simulink model "BLDC_Motor"  (R2018b)
settings: Solver=FixedStepDiscrete  StartTime=0.0  StopTime=2  MaxStep=1e-4  RelTol=1e-4
values from neighbouring files (symbols this model uses):
  A = 0    [control.m]
libraries: powerlib x10
settings Model: Creator=Nick  LastModifiedBy=Nick
settings SFSimCC: SimUseLocalCustomCode=off
settings RTWCC: RTWUseLocalCustomCode=off
settings CodeAppCC: StateflowObjectComments=on

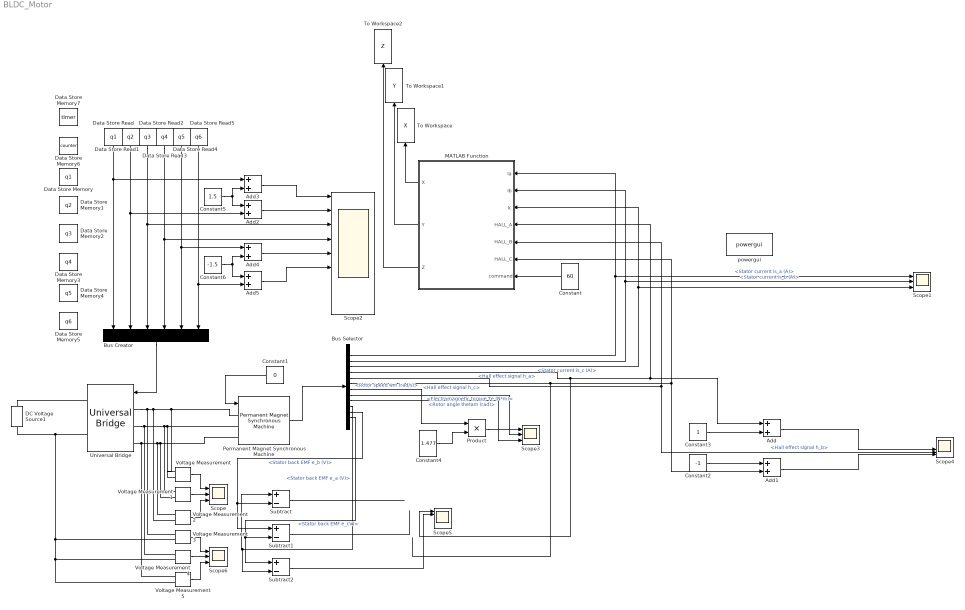
== system BLDC_Motor ==
  Add{,1..5} (6 alike) : Sum
  Bus Creator : BusCreator  Inputs=6
  Bus Selector : BusSelector  OutputSignals=Stator current is_a (A),Stator current is_b (A),Stator current is_c (A),Hall effect signal h_a,Hall effect signal h_b,Hall effect signal h_c,Rotor speed wm (rad/s),Electromagnetic torque Te (N*m),Rotor angle thetam (rad),Stator back EMF e_a (V),Stator back EMF e_b (V),Stator back EMF e_cV)
  Constant : Constant  Value=60
  Constant1 : Constant  Value=0
  Constant2 : Constant  Value=-1
  Constant3 : Constant
  Constant4 : Constant  Value=1.477
  Constant5 : Constant  Value=1.5
  Constant6 : Constant  Value=-1.5
  DC Voltage Source1 : powerlib/Electrical Sources/DC Voltage Source  Amplitude=48  Measurements=None
      settings: SourceProductName=Simscape Electrical
  Data Store Memory : DataStoreMemory  DataStoreName=q1  ReadBeforeWriteMsg=warning  WriteAfterWriteMsg=warning  WriteAfterReadMsg=warning  ShowAdditionalParam=off  OutDataTypeStr=double
  Data Store Memory1 : DataStoreMemory  DataStoreName=q2  ReadBeforeWriteMsg=warning  WriteAfterWriteMsg=warning  WriteAfterReadMsg=warning  ShowAdditionalParam=off  OutDataTypeStr=double
  Data Store Memory2 : DataStoreMemory  DataStoreName=q3  ReadBeforeWriteMsg=warning  WriteAfterWriteMsg=warning  WriteAfterReadMsg=warning  ShowAdditionalParam=off  OutDataTypeStr=double
  Data Store Memory3 : DataStoreMemory  DataStoreName=q4  ReadBeforeWriteMsg=warning  WriteAfterWriteMsg=warning  WriteAfterReadMsg=warning  ShowAdditionalParam=off  OutDataTypeStr=double
  Data Store Memory4 : DataStoreMemory  DataStoreName=q5  ReadBeforeWriteMsg=warning  WriteAfterWriteMsg=warning  WriteAfterReadMsg=warning  ShowAdditionalParam=off  OutDataTypeStr=double
  Data Store Memory5 : DataStoreMemory  DataStoreName=q6  ReadBeforeWriteMsg=warning  WriteAfterWriteMsg=warning  WriteAfterReadMsg=warning  ShowAdditionalParam=off  OutDataTypeStr=double
  Data Store Memory6 : DataStoreMemory  DataStoreName=counter  ReadBeforeWriteMsg=warning  WriteAfterWriteMsg=warning  WriteAfterReadMsg=warning  ShowAdditionalParam=off  OutDataTypeStr=double
  Data Store Memory7 : DataStoreMemory  DataStoreName=timer  ReadBeforeWriteMsg=warning  WriteAfterWriteMsg=warning  WriteAfterReadMsg=warning  ShowAdditionalParam=off  OutDataTypeStr=double
  Data Store Read : DataStoreRead  DataStoreName=q1
  Data Store Read1 : DataStoreRead  DataStoreName=q2
  Data Store Read2 : DataStoreRead  DataStoreName=q3
  Data Store Read3 : DataStoreRead  DataStoreName=q4
  Data Store Read4 : DataStoreRead  DataStoreName=q5
  Data Store Read5 : DataStoreRead  DataStoreName=q6
  MATLAB Function : MATLAB Function  TreatAsAtomicUnit=on
  Permanent Magnet Synchronous Machine : powerlib/Machines/Permanent Magnet Synchronous Machine  NbPhases=3  FluxDistribution=Trapezoidal  RotorType=Round  MechanicalLoad=Torque Tm  PresetModel=No  ShowDetailedParameters=on  MeasurementBus=off  Resistance=0.0485  Inductance=8.5e-3  dqInductances=[8.5e-3,8.5e-3]  La=0.000395  MachineConstant=Flux linkage established by magnets (V.s)  Flux=0.1194  VoltageCst=100.0283  TorqueCst=0.9552  Flat=120  Mechanical=[0.0027 0.0004924 4 0]  PolePairs=4  InitialConditions=[0,0, 0,0]  InitialConditions5ph=[0 0 0 0 0 0]  TsPowergui=0  TsBlock=-1  RefAngle=90 degrees behind phase A axis (modified Park)
  Product : Product
  Scope{,1,3,6} (4 alike) : Scope  NumInputPorts=3
  Scope2 : Scope  NumInputPorts=9
  Scope4 : Scope  NumInputPorts=6
  Scope5 : Scope  NumInputPorts=6
  Subtract : Sum  Inputs=+-
  Subtract1 : Sum  Inputs=+-
  Subtract2 : Sum  Inputs=+-
  To Workspace : ToWorkspace  VariableName=X  SaveFormat=Timeseries  SampleTime=-1
  To Workspace1 : ToWorkspace  VariableName=Y  SaveFormat=Timeseries  SampleTime=-1
  To Workspace2 : ToWorkspace  VariableName=Z  SaveFormat=Timeseries  SampleTime=-1
  Universal Bridge : powerlib/Power Electronics/Universal Bridge  Arms=3  SnubberResistance=1e5  SnubberCapacitance=inf  Device=MOSFET / Diodes  Ron=1e-3  Lon=0  ForwardVoltages="[  0  0  ]"  ForwardVoltage=0  GTOparameters=[ 10e-6 , 20e-6 ]  IGBTparameters=[ 1e-6 , 2e-6 ]  Measurements=None  Measurements_2=None  converterType=Rectifier
      settings: SourceProductName=Simscape Electrical
  Voltage Measurement{,1..5} (6 alike) : powerlib/Measurements/Voltage Measurement  PhasorSimulation=off  OutputType=Complex  PSBequivalent=0
      settings: SourceProductName=Simscape Electrical
  powergui : powerlib/powergui  Priority=1  SimulationMode=Discrete  SampleTime=50e-6  frequency=60  Iterations=50  frequencyindice=0  Pbase=100e6  ErrMax=1e-4  UnitsV=kV  UnitsW=MW  buscounter=0  FunctionMessages=off  echomessages=off  EnableUseOfTLC=off  CurrentSourceSwitches=off  DisableSnubberDevices=off  DisableRonSwitches=off  DisableVfSwitches=off  DisplayEquations=off  SolverType=Tustin/Backward Euler (TBE)  Interpol=off  ExternalGateDelay=off  methode=off  Ts=100  x0status=blocks  SPID=off  SwTol=0  HookPort=off  RestoreLinks=warning  ResistiveCurrentMeasurement=off  Frange=[0:2:500]  Ylog=off  Xlog=on  ShowGrid=off  save=off  variable=ZData  structure=0  ZoomFFT=off  StartTime=0.0  cycles=1  DisplayStyle=1  fundamental=60  FreqAxis=off  MaxFrequency=1000  frequencyindicesteady=1  RmsSteady=1  display=off
      settings: SourceProductName=Simscape Electrical
  wires:
  Permanent Magnet Synchronous Machine/1 -> Bus Selector/1
  Bus Selector/1 -> Scope1/1, MATLAB Function/1(Ia)  "<Stator current is_a (A)>"
  Constant/1 -> MATLAB Function/7(command)
  Bus Selector/2 -> Scope1/2, MATLAB Function/2(Ib)  "<Stator current is_b (A)>"
  Bus Selector/3 -> Scope1/3, MATLAB Function/3(Ic)  "<Stator current is_c (A)>"
  Bus Selector/5 -> Scope4/5, MATLAB Function/5(HALL_B)  "<Hall effect signal h_b>"
  Bus Selector/6 -> Add1/2, MATLAB Function/6(HALL_C)  "<Hall effect signal h_c>"
  Bus Selector/4 -> Scope5/1, Add/1, MATLAB Function/4(HALL_A)  "<Hall effect signal h_a>"
  Voltage Measurement/1 -> Scope/1
  Bus Creator/1 -> Universal Bridge/1
  Constant3/1 -> Add/2
  Constant2/1 -> Add1/1
  Add1/1 -> Scope4/6
  Add/1 -> Scope4/4
  Data Store Read/1 -> Bus Creator/1, Add3/1
  Data Store Read2/1 -> Scope2/3, Bus Creator/3
  Data Store Read3/1 -> Scope2/4, Bus Creator/4
  Data Store Read4/1 -> Add4/1, Bus Creator/5
  Constant1/1 -> Permanent Magnet Synchronous Machine/1
  Bus Selector/7 -> Product/1  "<Rotor speed wm (rad/s)>"
  Constant4/1 -> Product/2
  Product/1 -> Scope3/1
  Voltage Measurement4/1 -> Scope6/2
  Voltage Measurement3/1 -> Scope6/1
  Voltage Measurement5/1 -> Scope6/3
  Data Store Read1/1 -> Add2/2, Bus Creator/2
  Bus Selector/8 -> Scope3/2  "<Electromagnetic torque Te (N*m)>"
  Bus Selector/9 -> Scope3/3  "<Rotor angle thetam (rad)>"
  Voltage Measurement1/1 -> Scope/2
  Voltage Measurement2/1 -> Scope/3
  Add2/1 -> Scope2/2
  Constant5/1 -> Add2/1, Add3/2
  Add3/1 -> Scope2/1
  Add4/1 -> Scope2/5
  Add5/1 -> Scope2/6
  Constant6/1 -> Add5/1, Add4/2
  Data Store Read5/1 -> Add5/2, Bus Creator/6
  MATLAB Function/1(X) -> To Workspace/1
  MATLAB Function/2(Y) -> To Workspace1/1
  MATLAB Function/3(Z) -> To Workspace2/1
  Bus Selector/11 -> Subtract/2, Subtract1/1  "<Stator back EMF e_b (V)>"
  Subtract/1 -> ?
  Bus Selector/12 -> Subtract2/1, Subtract1/2  "<Stator back EMF e_cV)>"
  Bus Selector/10 -> Subtract2/2, Subtract/1  "<Stator back EMF e_a (V)>"
  Subtract1/1 -> ?
  Subtract2/1 -> Scope5/2
  connections:
  Universal Bridge/LConn1 -- Voltage Measurement3/LConn1 -- Voltage Measurement2/LConn2 -- Permanent Magnet Synchronous Machine/LConn1 -- Voltage Measurement/LConn1
  Universal Bridge/LConn2 -- Voltage Measurement4/LConn1 -- Voltage Measurement1/LConn1 -- Permanent Magnet Synchronous Machine/LConn2 -- Voltage Measurement/LConn2
  Universal Bridge/LConn3 -- Voltage Measurement5/LConn1 -- Voltage Measurement2/LConn1 -- Permanent Magnet Synchronous Machine/LConn3 -- Voltage Measurement1/LConn2
  Universal Bridge/RConn1 -- DC Voltage Source1/RConn1
  Universal Bridge/RConn2 -- Voltage Measurement5/LConn2 -- Voltage Measurement4/LConn2 -- Voltage Measurement3/LConn2 -- DC Voltage Source1/LConn1

== matlab function BLDC_Motor/MATLAB Function ==
  settings: updateMethod=DISCRETE  sampleTime=50e-7
  data: Ia input size=1; Ib input size=1; Ic input size=1; HALL_A input; HALL_B input; HALL_C input size=1; command input size=1; q1 data_store_memory; q2 data_store_memory; q3 data_store_memory; q4 data_store_memory; q5 data_store_memory; q6 data_store_memory; counter data_store_memory; timer data_store_memory; X output; Y output; Z output
function [X,Y,Z] = control(Ia,Ib,Ic,HALL_A,HALL_B,HALL_C,command)
global q1 
global q2 
global q3 
global q4 
global q5 
global q6
global counter
X = (2*Ia - Ib - Ic)*(1/sqrt(6));
Y = (Ib - Ic)*(1/sqrt(2));
Z = (Ia + Ib + Ic)*(1/sqrt(3));

counter = counter + 1;
if counter <= command
    if HALL_A && ~HALL_B && HALL_C
        q1 = 1;
        q2 = 0;
        q3 = 0;
        q4 = 1;
        q5 = 1;
        q6 = 0;

    elseif HALL_A && ~HALL_B && ~HALL_C
        q1 = 1;
        q2 = 0;
        q3 = 0;
        q4 = 1;
        q5 = 0;
        q6 = 1;

    elseif HALL_A && HALL_B && ~HALL_C
        q1 = 1;
        q2 = 0;
        q3 = 1;
        q4 = 0;
        q5 = 0;
        q6 = 1;

    elseif ~HALL_A && HALL_B && ~HALL_C
        q1 = 0;
        q2 = 1;
        q3 = 1;
        q4 = 0;
        q5 = 0;
        q6 = 1;

    elseif ~HALL_A && HALL_B && HALL_C
        q1 = 0;
        q2 = 1;
        q3 = 1;
        q4 = 0;
        q5 = 1;
        q6 = 0; 

    elseif ~HALL_A && ~HALL_B && HALL_C
        q1 = 0;
        q2 = 1;
        q3 = 0;
        q4 = 1;
        q5 = 1;
        q6 = 0;
    end
else
    q1 = 0;
    q2 = 0;
    q3 = 0;
    q4 = 0;
    q5 = 0;
    q6 = 0;
end
if counter >= 100
    counter = 0;
end
